simulink model "sldemo_bangbang"  (R2019b)
settings: Solver=ode23  StartTime=0.0  StopTime=100  MaxStep=0.1  RelTol=1e-6  AbsTol=1e-6
libraries: simulink x1
Description:
  | State Events
  | 
  | This example shows how to handle state events.  Run the simulation and see the
  | phase plane plot, where the state x1 is along the X-axis and the state x2 is along
  | the Y-axis.
settings Model: ExtModeAutoUpdateStatusClock=off  Creator=The MathWorks, Inc.  LastModifiedBy=bhisma
settings SolverCC: AutoScaleAbsTol=off
settings DataIOCC: ExternalInput=[]  InitialState=[]  SaveFormat=Array  SaveOutput=off  SignalLogging=off  SaveTime=off  ReturnWorkspaceOutputs=off  StateSaveName=x  TimeSaveName=t
settings OptimizationCC: InitFltsAndDblsToZero=on  LifeSpan=inf  BufferReusableBoundary=off
settings DebuggingCC: SaveWithParameterizedLinksMsg=none  UnderspecifiedInitializationDetection=Classic  MergeDetectMultiDrivingBlocksExec=none  SignalResolutionControl=TryResolveAllWithWarning  MultiTaskDSMMsg=warning  MultiTaskCondExecSysMsg=none  FcnCallInpInsideContextMsg=warning  BusObjectLabelMismatch=none  StateNameClashWarn=warning  SFUnexpectedBacktrackingDiag=warning  SFNoUnconditionalDefaultTransitionDiag=warning  SFExecutionAtInitializationDiag=none  ArithmeticOperatorsInVariantConditions=warning
settings HardwareCC: ProdBitPerPointer=32  ProdBitPerSizeT=32  ProdBitPerPtrDiffT=32  ProdLargestAtomicFloat=None  ProdIntDivRoundTo=Undefined  ProdEndianess=Unspecified  ProdWordSize=32  ProdHWDeviceType=32-bit Generic  TargetUnknown=on
settings ModelReferenceCC: PropagateSignalLabelsOutOfModel=off
settings SFSimCC: SimUseLocalCustomCode=off
settings RTWCC: Description=Generic Real-Time Target  RTWUseLocalCustomCode=off
settings CodeAppCC: StateflowObjectComments=on
settings GRTTargetCC: TargetFcnLib=ansi_tfl_tmw.mat  TargetLangStandard=C89/C90 (ANSI)  GeneratePreprocessorConditionals=Disable all  CombineOutputUpdateFcns=off  GRTInterface=on
settings ConfigComp: CovMetricSettings=dw  CovHtmlReporting=on  CovSaveCumulativeToWorkspaceVar=on  CovSaveSingleToWorkspaceVar=on  CovExternalEMLEnable=off

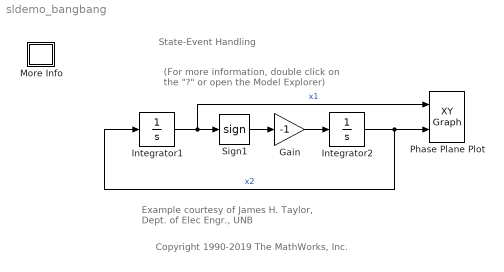
== system sldemo_bangbang ==
  note: State-Event Handling
  note: Example courtesy of James H. Taylor,
      | Dept. of Elec Engr., UNB
  note: (For more information, double click on
      | the "?" or open the Model Explorer)
  note: Copyright 1990-2019 The MathWorks, Inc.
  Gain : Gain  Gain=-1  SaturateOnIntegerOverflow=on  OutDataTypeStr=Inherit: Same as input  ParamDataTypeStr=Inherit: Same as input
  Integrator1 : Integrator  InitialCondition=0.25
  Integrator2 : Integrator  InitialCondition=0.25
  More Info : Subsystem
      settings: OpenFcn=showExample('simulink_general/sldemo_bangbangExample')
      mask Display: disp('?')
  Phase Plane Plot : simulink/Sinks/XY Graph  xmin=-0.3  xmax=0.3  ymin=-0.8  ymax=0.8  st=-1
  Sign1 : Signum
  wires:
  Integrator2/1 -> Integrator1/1, Phase Plane Plot/2  "x2"
  Integrator1/1 -> Phase Plane Plot/1, Sign1/1  "x1"
  Sign1/1 -> Gain/1
  Gain/1 -> Integrator2/1

== system sldemo_bangbang/More Info ==
